simulink model "controllerTester"  (R2015b)
settings: Solver=FixedStepDiscrete  StartTime=0.0  StopTime=10.0  RelTol=1e-3
libraries: simulink x1, fuzblock x1
settings Model: Creator=sprinkle  LastModifiedBy=sprinkle

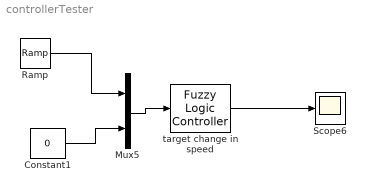
== system controllerTester ==
  Constant1 : Constant  Value=0
  Mux5 : Mux  Inputs=2
  Ramp : simulink/Sources/Ramp  slope=1  start=0  X0=5
  Scope6 : Scope
  target change in speed : fuzblock/Fuzzy Logic  Controller  fis='spring2.fis'
  wires:
  Ramp/1 -> Mux5/1
  Constant1/1 -> Mux5/2
  Mux5/1 -> target change in speed/1
  target change in speed/1 -> Scope6/1
